simulink model "motorsPID"  (R2015a)
settings: Solver=ode45  StartTime=0.0  StopTime=Tsim  RelTol=1e-3
values from neighbouring files (symbols this model uses):
  b = 0.1    [AjusteC.m]    (also in AjusteC2.m; AjusteCVaryReal.m; GenPath.m = m*(2.0*pi/L); GenPath2.m = m*(2.0*pi/L))
  d = 0.4    [AjusteC.m]    (also in AjusteC2.m; AjusteCVaryReal.m; simula_robo.m)
  J = 0.01    [AjusteC.m]    (also in AjusteC2.m; AjusteCVaryReal.m; simula_robo.m)
  Kd = 0    [AjusteC.m]    (also in AjusteC2.m; AjusteCVaryReal.m; simula_robo.m)
  Ke = 0.08    [AjusteC.m]    (also in AjusteC2.m; AjusteCVaryReal.m; simula_robo.m)
  Ki = 10.0    (= 10)    [AjusteC.m]    (also in AjusteC2.m; AjusteCVaryReal.m; simula_robo.m)
  Kp = 5    [AjusteC.m]    (also in AjusteC2.m; AjusteCVaryReal.m; simula_robo.m)
  L = 0.5    [AjusteC.m]    (also in AjusteC2.m; AjusteCVaryReal.m; GenPath.m = input('Entre o comprimento m�ximo: '); GenPath2.m = input('Entre o comprimento m�ximo: '))
  Res = 1    [AjusteC.m]    (also in AjusteC2.m; AjusteCVaryReal.m; simula_robo.m)
  thetai = 0    [AjusteC.m]    (also in AjusteC2.m; AjusteCVaryReal.m; simula_robo.m = 1.57079632679)
  Ts = 0.1    [AjusteC.m]    (also in AjusteC2.m; AjusteCVaryReal.m; GenPath.m; GenPath2.m)
  vmax = 0.8    [AjusteC.m]    (also in AjusteC2.m; AjusteCVaryReal.m; simula_robo.m)
  vmin = -vmax    (= -0.8)    [AjusteC.m]    (also in AjusteC2.m; AjusteCVaryReal.m; simula_robo.m)
  wmax = 0.8    [AjusteC.m]    (also in AjusteC2.m; AjusteCVaryReal.m; simula_robo.m)
  wmin = -wmax    (= -0.8)    [AjusteC.m]    (also in AjusteC2.m; AjusteCVaryReal.m; simula_robo.m)
  xi = 0    [AjusteC.m]    (also in AjusteC2.m; AjusteCVaryReal.m = 1; simula_robo.m)
  yi = 0    [AjusteC.m]    (also in AjusteC2.m; AjusteCVaryReal.m = -3; simula_robo.m = -0.5)
libraries: simulink_extras x6, simulink x6
settings Model: Creator=Thiago  LastModifiedBy=Thiago

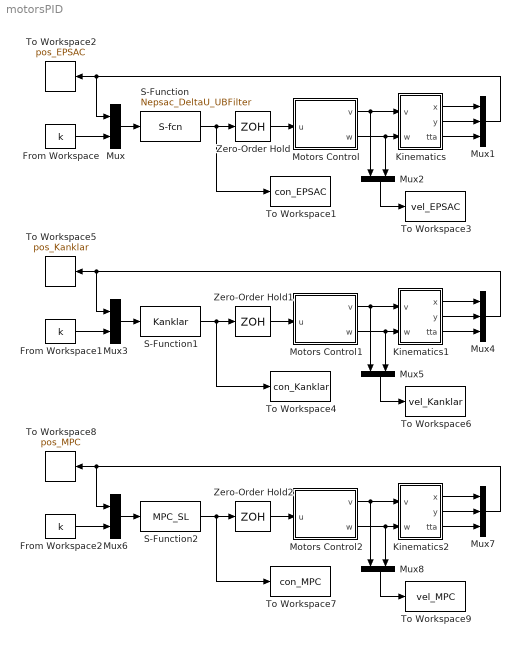
== system motorsPID ==
  From Workspace : FromWorkspace  VariableName=k  SampleTime=Ts
  From Workspace1 : FromWorkspace  VariableName=k  SampleTime=Ts
  From Workspace2 : FromWorkspace  VariableName=k  SampleTime=Ts
  Kinematics : Subsystem
  Kinematics1 : Subsystem
  Kinematics2 : Subsystem
  Motors Control : Subsystem
  Motors Control1 : Subsystem
  Motors Control2 : Subsystem
  Mux{,2..3,5..6,8} (6 alike) : Mux  Inputs=2
  Mux1 : Mux  Inputs=3
  Mux4 : Mux  Inputs=3
  Mux7 : Mux  Inputs=3
  S-Function : S-Function  FunctionName=Nepsac_DeltaU_UBFilter
  S-Function1 : S-Function  FunctionName=Kanklar
  S-Function2 : S-Function  FunctionName=MPC_SL
  To Workspace1 : ToWorkspace  VariableName=con_EPSAC  SaveFormat=Structure With Time  SampleTime=Ts
  To Workspace2 : ToWorkspace  VariableName=pos_EPSAC  SaveFormat=Structure With Time  SampleTime=Ts
  To Workspace3 : ToWorkspace  VariableName=vel_EPSAC  SaveFormat=Structure With Time  SampleTime=Ts
  To Workspace4 : ToWorkspace  VariableName=con_Kanklar  SaveFormat=Structure With Time  SampleTime=Ts
  To Workspace5 : ToWorkspace  VariableName=pos_Kanklar  SaveFormat=Structure With Time  SampleTime=Ts
  To Workspace6 : ToWorkspace  VariableName=vel_Kanklar  SaveFormat=Structure With Time  SampleTime=Ts
  To Workspace7 : ToWorkspace  VariableName=con_MPC  SaveFormat=Structure With Time  SampleTime=Ts
  To Workspace8 : ToWorkspace  VariableName=pos_MPC  SaveFormat=Structure With Time  SampleTime=Ts
  To Workspace9 : ToWorkspace  VariableName=vel_MPC  SaveFormat=Structure With Time  SampleTime=Ts
  Zero-Order Hold : ZeroOrderHold  SampleTime=Ts
  Zero-Order Hold1 : ZeroOrderHold  SampleTime=Ts
  Zero-Order Hold2 : ZeroOrderHold  SampleTime=Ts
  wires:
  S-Function/1 -> Zero-Order Hold/1, To Workspace1/1
  Motors Control/1(v) -> Kinematics/1(v), Mux2/1
  Motors Control/2(w) -> Kinematics/2(w), Mux2/2
  Kinematics/1(x) -> Mux1/1
  Kinematics/2(y) -> Mux1/2
  Kinematics/3(tta) -> Mux1/3
  Mux/1 -> S-Function/1
  From Workspace/1 -> Mux/2
  Mux1/1 -> Mux/1, To Workspace2/1
  Mux2/1 -> To Workspace3/1
  Zero-Order Hold/1 -> Motors Control/1(u)
  S-Function1/1 -> Zero-Order Hold1/1, To Workspace4/1
  Motors Control1/1(v) -> Kinematics1/1(v), Mux5/1
  Motors Control1/2(w) -> Kinematics1/2(w), Mux5/2
  Kinematics1/1(x) -> Mux4/1
  Kinematics1/2(y) -> Mux4/2
  Kinematics1/3(tta) -> Mux4/3
  Mux3/1 -> S-Function1/1
  From Workspace1/1 -> Mux3/2
  Mux4/1 -> Mux3/1, To Workspace5/1
  Mux5/1 -> To Workspace6/1
  Zero-Order Hold1/1 -> Motors Control1/1(u)
  S-Function2/1 -> Zero-Order Hold2/1, To Workspace7/1
  Motors Control2/1(v) -> Kinematics2/1(v), Mux8/1
  Motors Control2/2(w) -> Kinematics2/2(w), Mux8/2
  Kinematics2/1(x) -> Mux7/1
  Kinematics2/2(y) -> Mux7/2
  Kinematics2/3(tta) -> Mux7/3
  Mux6/1 -> S-Function2/1
  From Workspace2/1 -> Mux6/2
  Mux7/1 -> Mux6/1, To Workspace8/1
  Mux8/1 -> To Workspace9/1
  Zero-Order Hold2/1 -> Motors Control2/1(u)

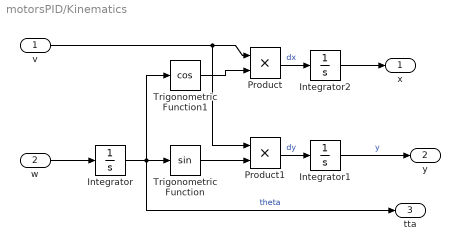
== system motorsPID/Kinematics ==
  v : Inport
  w : Inport  Port=2
  Integrator : Integrator  InitialCondition=thetai
  Integrator1 : Integrator  InitialCondition=yi
  Integrator2 : Integrator  InitialCondition=xi
  Product : Product
  Product1 : Product
  Trigonometric Function : Trigonometry
  Trigonometric Function1 : Trigonometry  Operator=cos
  x : Outport
  y : Outport  Port=2
  tta : Outport  Port=3
  wires:
  v/1 -> Product1/1, Product/1
  Trigonometric Function1/1 -> Product/2
  Product/1 -> Integrator2/1  "dx"
  Integrator/1 -> tta/1, Trigonometric Function1/1, Trigonometric Function/1  "theta"
  Integrator1/1 -> y/1  "y"
  Product1/1 -> Integrator1/1  "dy"
  Trigonometric Function/1 -> Product1/2
  Integrator2/1 -> x/1
  w/1 -> Integrator/1

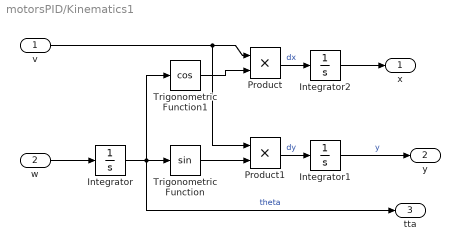
== system motorsPID/Kinematics1 ==
  v : Inport
  w : Inport  Port=2
  Integrator : Integrator  InitialCondition=thetai
  Integrator1 : Integrator  InitialCondition=yi
  Integrator2 : Integrator  InitialCondition=xi
  Product : Product
  Product1 : Product
  Trigonometric Function : Trigonometry
  Trigonometric Function1 : Trigonometry  Operator=cos
  x : Outport
  y : Outport  Port=2
  tta : Outport  Port=3
  wires:
  v/1 -> Product1/1, Product/1
  Trigonometric Function1/1 -> Product/2
  Product/1 -> Integrator2/1  "dx"
  Integrator/1 -> tta/1, Trigonometric Function1/1, Trigonometric Function/1  "theta"
  Integrator1/1 -> y/1  "y"
  Product1/1 -> Integrator1/1  "dy"
  Trigonometric Function/1 -> Product1/2
  Integrator2/1 -> x/1
  w/1 -> Integrator/1

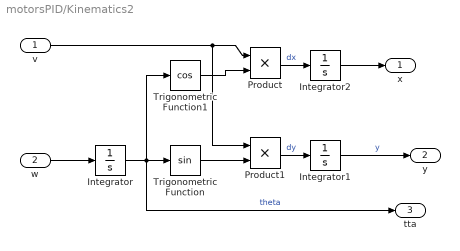
== system motorsPID/Kinematics2 ==
  v : Inport
  w : Inport  Port=2
  Integrator : Integrator  InitialCondition=thetai
  Integrator1 : Integrator  InitialCondition=yi
  Integrator2 : Integrator  InitialCondition=xi
  Product : Product
  Product1 : Product
  Trigonometric Function : Trigonometry
  Trigonometric Function1 : Trigonometry  Operator=cos
  x : Outport
  y : Outport  Port=2
  tta : Outport  Port=3
  wires:
  v/1 -> Product1/1, Product/1
  Trigonometric Function1/1 -> Product/2
  Product/1 -> Integrator2/1  "dx"
  Integrator/1 -> tta/1, Trigonometric Function1/1, Trigonometric Function/1  "theta"
  Integrator1/1 -> y/1  "y"
  Product1/1 -> Integrator1/1  "dy"
  Trigonometric Function/1 -> Product1/2
  Integrator2/1 -> x/1
  w/1 -> Integrator/1

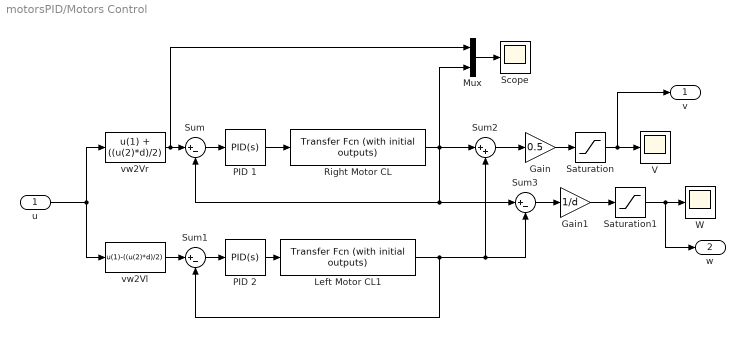
== system motorsPID/Motors Control ==
  u : Inport
  Gain : Gain  Gain=0.5
  Gain1 : Gain  Gain=1/d
  Left Motor CL1 : simulink_extras/Additional Linear/Transfer Fcn (with initial outputs)  N=[Ke]  D="[J*L  (J*Res+b*L) (b*Res+Ke^2)]"  Y0=0  U0=0
  Mux : Mux  Inputs=2
  PID 1 : simulink/Continuous/PID Controller  Controller=PID  TimeDomain=Continuous-time  SampleTime=-1  IntegratorMethod=Forward Euler  FilterMethod=Forward Euler  Form=Parallel  UseFilter=on  ControllerParametersSource=internal  P=Kp  I=Ki  D=Kd  N=100  InitialConditionSource=internal  InitialConditionForIntegrator=0  InitialConditionForFilter=0  ExternalReset=none  LimitOutput=off  UpperSaturationLimit=inf  LowerSaturationLimit=-inf  LinearizeAsGain=on  AntiWindupMode=none  Kb=1  TrackingMode=off  Kt=1  PParamMin=[]  PParamMax=[]  IParamMin=[]  IParamMax=[]  DParamMin=[]  DParamMax=[]  NParamMin=[]  NParamMax=[]  KbParamMin=[]  KbParamMax=[]  KtParamMin=[]  KtParamMax=[]  POutMin=[]  POutMax=[]  IOutMin=[]  IOutMax=[]  DOutMin=[]  DOutMax=[]  NOutMin=[]  NOutMax=[]  KbOutMin=[]  KbOutMax=[]  KtOutMin=[]  KtOutMax=[]  IntegratorOutMin=[]  IntegratorOutMax=[]  FilterOutMin=[]  FilterOutMax=[]  SumOutMin=[]  SumOutMax=[]  SumI1OutMin=[]  SumI1OutMax=[]  SumI2OutMin=[]  SumI2OutMax=[]  SumI3OutMin=[]  SumI3OutMax=[]  SumDOutMin=[]  SumDOutMax=[]  SaturationOutMin=[]  SaturationOutMax=[]  IntegratorContinuousStateAttributes=''  IntegratorStateMustResolveToSignalObject=off  IntegratorRTWStateStorageClass=Auto  FilterContinuousStateAttributes=''  FilterStateMustResolveToSignalObject=off  FilterRTWStateStorageClass=Auto  DifferentiatorICPrevScaledInput=0  DifferentiatorOutMin=[]  DifferentiatorOutMax=[]
  PID 2 : simulink/Continuous/PID Controller  Controller=PID  TimeDomain=Continuous-time  SampleTime=-1  IntegratorMethod=Forward Euler  FilterMethod=Forward Euler  Form=Parallel  UseFilter=on  ControllerParametersSource=internal  P=Kp  I=Ki  D=Kd  N=100  InitialConditionSource=internal  InitialConditionForIntegrator=0  InitialConditionForFilter=0  ExternalReset=none  LimitOutput=off  UpperSaturationLimit=inf  LowerSaturationLimit=-inf  LinearizeAsGain=on  AntiWindupMode=none  Kb=1  TrackingMode=off  Kt=1  PParamMin=[]  PParamMax=[]  IParamMin=[]  IParamMax=[]  DParamMin=[]  DParamMax=[]  NParamMin=[]  NParamMax=[]  KbParamMin=[]  KbParamMax=[]  KtParamMin=[]  KtParamMax=[]  POutMin=[]  POutMax=[]  IOutMin=[]  IOutMax=[]  DOutMin=[]  DOutMax=[]  NOutMin=[]  NOutMax=[]  KbOutMin=[]  KbOutMax=[]  KtOutMin=[]  KtOutMax=[]  IntegratorOutMin=[]  IntegratorOutMax=[]  FilterOutMin=[]  FilterOutMax=[]  SumOutMin=[]  SumOutMax=[]  SumI1OutMin=[]  SumI1OutMax=[]  SumI2OutMin=[]  SumI2OutMax=[]  SumI3OutMin=[]  SumI3OutMax=[]  SumDOutMin=[]  SumDOutMax=[]  SaturationOutMin=[]  SaturationOutMax=[]  IntegratorContinuousStateAttributes=''  IntegratorStateMustResolveToSignalObject=off  IntegratorRTWStateStorageClass=Auto  FilterContinuousStateAttributes=''  FilterStateMustResolveToSignalObject=off  FilterRTWStateStorageClass=Auto  DifferentiatorICPrevScaledInput=0  DifferentiatorOutMin=[]  DifferentiatorOutMax=[]
  Right Motor CL : simulink_extras/Additional Linear/Transfer Fcn (with initial outputs)  N=[Ke]  D="[J*L  (J*Res+b*L) (b*Res+Ke^2)]"  Y0=0  U0=0
  Saturation : Saturate  UpperLimit=vmax  LowerLimit=vmin
  Saturation1 : Saturate  UpperLimit=wmax  LowerLimit=wmin
  Scope : Scope
      settings: SaveName=ScopeData3
  Sum : Sum  Inputs=|+-
  Sum1 : Sum  Inputs=|+-
  Sum2 : Sum  Inputs=|++
  Sum3 : Sum  Inputs=|+-
  V : Scope
  W : Scope
      settings: SaveName=ScopeData2
  vw2Vl : Fcn  Expr=u(1)-((u(2)*d)/2)
  vw2Vr : Fcn  Expr=u(1) + ((u(2)*d)/2)
  v : Outport
  w : Outport  Port=2
  wires:
  u/1 -> vw2Vr/1, vw2Vl/1
  PID 1/1 -> Right Motor CL/1
  Sum/1 -> PID 1/1
  PID 2/1 -> Left Motor CL1/1
  Sum1/1 -> PID 2/1
  vw2Vl/1 -> Sum1/1
  Left Motor CL1/1 -> Sum3/2, Sum2/2, Sum1/2
  vw2Vr/1 -> Mux/1, Sum/1
  Right Motor CL/1 -> Mux/2, Sum2/1, Sum3/1, Sum/2
  Sum2/1 -> Gain/1
  Sum3/1 -> Gain1/1
  Mux/1 -> Scope/1
  Gain/1 -> Saturation/1
  Saturation/1 -> v/1, V/1
  Gain1/1 -> Saturation1/1
  Saturation1/1 -> W/1, w/1

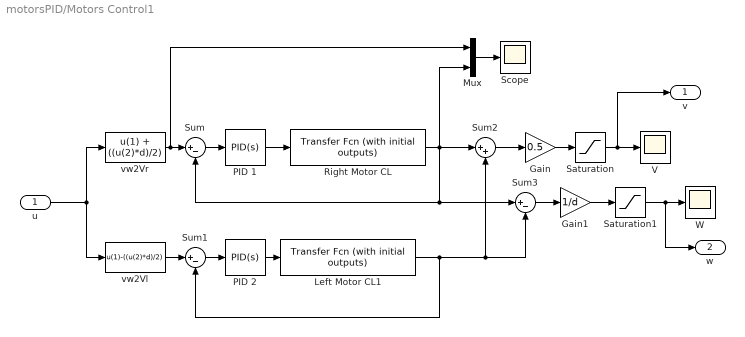
== system motorsPID/Motors Control1 ==
  u : Inport
  Gain : Gain  Gain=0.5
  Gain1 : Gain  Gain=1/d
  Left Motor CL1 : simulink_extras/Additional Linear/Transfer Fcn (with initial outputs)  N=[Ke]  D="[J*L  (J*Res+b*L) (b*Res+Ke^2)]"  Y0=0  U0=0
  Mux : Mux  Inputs=2
  PID 1 : simulink/Continuous/PID Controller  Controller=PID  TimeDomain=Continuous-time  SampleTime=-1  IntegratorMethod=Forward Euler  FilterMethod=Forward Euler  Form=Parallel  UseFilter=on  ControllerParametersSource=internal  P=Kp  I=Ki  D=Kd  N=100  InitialConditionSource=internal  InitialConditionForIntegrator=0  InitialConditionForFilter=0  ExternalReset=none  LimitOutput=off  UpperSaturationLimit=inf  LowerSaturationLimit=-inf  LinearizeAsGain=on  AntiWindupMode=none  Kb=1  TrackingMode=off  Kt=1  PParamMin=[]  PParamMax=[]  IParamMin=[]  IParamMax=[]  DParamMin=[]  DParamMax=[]  NParamMin=[]  NParamMax=[]  KbParamMin=[]  KbParamMax=[]  KtParamMin=[]  KtParamMax=[]  POutMin=[]  POutMax=[]  IOutMin=[]  IOutMax=[]  DOutMin=[]  DOutMax=[]  NOutMin=[]  NOutMax=[]  KbOutMin=[]  KbOutMax=[]  KtOutMin=[]  KtOutMax=[]  IntegratorOutMin=[]  IntegratorOutMax=[]  FilterOutMin=[]  FilterOutMax=[]  SumOutMin=[]  SumOutMax=[]  SumI1OutMin=[]  SumI1OutMax=[]  SumI2OutMin=[]  SumI2OutMax=[]  SumI3OutMin=[]  SumI3OutMax=[]  SumDOutMin=[]  SumDOutMax=[]  SaturationOutMin=[]  SaturationOutMax=[]  IntegratorContinuousStateAttributes=''  IntegratorStateMustResolveToSignalObject=off  IntegratorRTWStateStorageClass=Auto  FilterContinuousStateAttributes=''  FilterStateMustResolveToSignalObject=off  FilterRTWStateStorageClass=Auto  DifferentiatorICPrevScaledInput=0  DifferentiatorOutMin=[]  DifferentiatorOutMax=[]
  PID 2 : simulink/Continuous/PID Controller  Controller=PID  TimeDomain=Continuous-time  SampleTime=-1  IntegratorMethod=Forward Euler  FilterMethod=Forward Euler  Form=Parallel  UseFilter=on  ControllerParametersSource=internal  P=Kp  I=Ki  D=Kd  N=100  InitialConditionSource=internal  InitialConditionForIntegrator=0  InitialConditionForFilter=0  ExternalReset=none  LimitOutput=off  UpperSaturationLimit=inf  LowerSaturationLimit=-inf  LinearizeAsGain=on  AntiWindupMode=none  Kb=1  TrackingMode=off  Kt=1  PParamMin=[]  PParamMax=[]  IParamMin=[]  IParamMax=[]  DParamMin=[]  DParamMax=[]  NParamMin=[]  NParamMax=[]  KbParamMin=[]  KbParamMax=[]  KtParamMin=[]  KtParamMax=[]  POutMin=[]  POutMax=[]  IOutMin=[]  IOutMax=[]  DOutMin=[]  DOutMax=[]  NOutMin=[]  NOutMax=[]  KbOutMin=[]  KbOutMax=[]  KtOutMin=[]  KtOutMax=[]  IntegratorOutMin=[]  IntegratorOutMax=[]  FilterOutMin=[]  FilterOutMax=[]  SumOutMin=[]  SumOutMax=[]  SumI1OutMin=[]  SumI1OutMax=[]  SumI2OutMin=[]  SumI2OutMax=[]  SumI3OutMin=[]  SumI3OutMax=[]  SumDOutMin=[]  SumDOutMax=[]  SaturationOutMin=[]  SaturationOutMax=[]  IntegratorContinuousStateAttributes=''  IntegratorStateMustResolveToSignalObject=off  IntegratorRTWStateStorageClass=Auto  FilterContinuousStateAttributes=''  FilterStateMustResolveToSignalObject=off  FilterRTWStateStorageClass=Auto  DifferentiatorICPrevScaledInput=0  DifferentiatorOutMin=[]  DifferentiatorOutMax=[]
  Right Motor CL : simulink_extras/Additional Linear/Transfer Fcn (with initial outputs)  N=[Ke]  D="[J*L  (J*Res+b*L) (b*Res+Ke^2)]"  Y0=0  U0=0
  Saturation : Saturate  UpperLimit=vmax  LowerLimit=vmin
  Saturation1 : Saturate  UpperLimit=wmax  LowerLimit=wmin
  Scope : Scope
      settings: SaveName=ScopeData3
  Sum : Sum  Inputs=|+-
  Sum1 : Sum  Inputs=|+-
  Sum2 : Sum  Inputs=|++
  Sum3 : Sum  Inputs=|+-
  V : Scope
  W : Scope
      settings: SaveName=ScopeData2
  vw2Vl : Fcn  Expr=u(1)-((u(2)*d)/2)
  vw2Vr : Fcn  Expr=u(1) + ((u(2)*d)/2)
  v : Outport
  w : Outport  Port=2
  wires:
  u/1 -> vw2Vr/1, vw2Vl/1
  PID 1/1 -> Right Motor CL/1
  Sum/1 -> PID 1/1
  PID 2/1 -> Left Motor CL1/1
  Sum1/1 -> PID 2/1
  vw2Vl/1 -> Sum1/1
  Left Motor CL1/1 -> Sum3/2, Sum2/2, Sum1/2
  vw2Vr/1 -> Mux/1, Sum/1
  Right Motor CL/1 -> Mux/2, Sum2/1, Sum3/1, Sum/2
  Sum2/1 -> Gain/1
  Sum3/1 -> Gain1/1
  Mux/1 -> Scope/1
  Gain/1 -> Saturation/1
  Saturation/1 -> v/1, V/1
  Gain1/1 -> Saturation1/1
  Saturation1/1 -> W/1, w/1

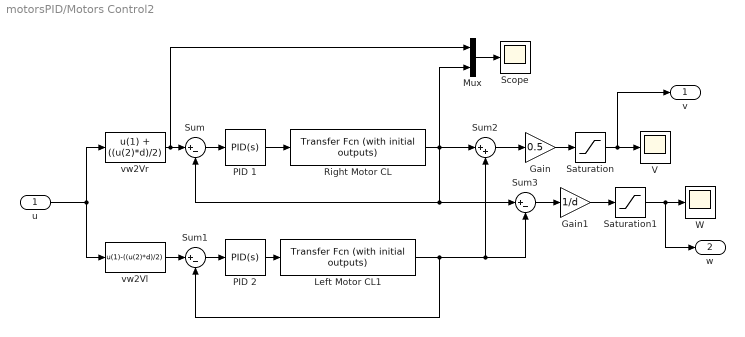
== system motorsPID/Motors Control2 ==
  u : Inport
  Gain : Gain  Gain=0.5
  Gain1 : Gain  Gain=1/d
  Left Motor CL1 : simulink_extras/Additional Linear/Transfer Fcn (with initial outputs)  N=[Ke]  D="[J*L  (J*Res+b*L) (b*Res+Ke^2)]"  Y0=0  U0=0
  Mux : Mux  Inputs=2
  PID 1 : simulink/Continuous/PID Controller  Controller=PID  TimeDomain=Continuous-time  SampleTime=-1  IntegratorMethod=Forward Euler  FilterMethod=Forward Euler  Form=Parallel  UseFilter=on  ControllerParametersSource=internal  P=Kp  I=Ki  D=Kd  N=100  InitialConditionSource=internal  InitialConditionForIntegrator=0  InitialConditionForFilter=0  ExternalReset=none  LimitOutput=off  UpperSaturationLimit=inf  LowerSaturationLimit=-inf  LinearizeAsGain=on  AntiWindupMode=none  Kb=1  TrackingMode=off  Kt=1  PParamMin=[]  PParamMax=[]  IParamMin=[]  IParamMax=[]  DParamMin=[]  DParamMax=[]  NParamMin=[]  NParamMax=[]  KbParamMin=[]  KbParamMax=[]  KtParamMin=[]  KtParamMax=[]  POutMin=[]  POutMax=[]  IOutMin=[]  IOutMax=[]  DOutMin=[]  DOutMax=[]  NOutMin=[]  NOutMax=[]  KbOutMin=[]  KbOutMax=[]  KtOutMin=[]  KtOutMax=[]  IntegratorOutMin=[]  IntegratorOutMax=[]  FilterOutMin=[]  FilterOutMax=[]  SumOutMin=[]  SumOutMax=[]  SumI1OutMin=[]  SumI1OutMax=[]  SumI2OutMin=[]  SumI2OutMax=[]  SumI3OutMin=[]  SumI3OutMax=[]  SumDOutMin=[]  SumDOutMax=[]  SaturationOutMin=[]  SaturationOutMax=[]  IntegratorContinuousStateAttributes=''  IntegratorStateMustResolveToSignalObject=off  IntegratorRTWStateStorageClass=Auto  FilterContinuousStateAttributes=''  FilterStateMustResolveToSignalObject=off  FilterRTWStateStorageClass=Auto  DifferentiatorICPrevScaledInput=0  DifferentiatorOutMin=[]  DifferentiatorOutMax=[]
  PID 2 : simulink/Continuous/PID Controller  Controller=PID  TimeDomain=Continuous-time  SampleTime=-1  IntegratorMethod=Forward Euler  FilterMethod=Forward Euler  Form=Parallel  UseFilter=on  ControllerParametersSource=internal  P=Kp  I=Ki  D=Kd  N=100  InitialConditionSource=internal  InitialConditionForIntegrator=0  InitialConditionForFilter=0  ExternalReset=none  LimitOutput=off  UpperSaturationLimit=inf  LowerSaturationLimit=-inf  LinearizeAsGain=on  AntiWindupMode=none  Kb=1  TrackingMode=off  Kt=1  PParamMin=[]  PParamMax=[]  IParamMin=[]  IParamMax=[]  DParamMin=[]  DParamMax=[]  NParamMin=[]  NParamMax=[]  KbParamMin=[]  KbParamMax=[]  KtParamMin=[]  KtParamMax=[]  POutMin=[]  POutMax=[]  IOutMin=[]  IOutMax=[]  DOutMin=[]  DOutMax=[]  NOutMin=[]  NOutMax=[]  KbOutMin=[]  KbOutMax=[]  KtOutMin=[]  KtOutMax=[]  IntegratorOutMin=[]  IntegratorOutMax=[]  FilterOutMin=[]  FilterOutMax=[]  SumOutMin=[]  SumOutMax=[]  SumI1OutMin=[]  SumI1OutMax=[]  SumI2OutMin=[]  SumI2OutMax=[]  SumI3OutMin=[]  SumI3OutMax=[]  SumDOutMin=[]  SumDOutMax=[]  SaturationOutMin=[]  SaturationOutMax=[]  IntegratorContinuousStateAttributes=''  IntegratorStateMustResolveToSignalObject=off  IntegratorRTWStateStorageClass=Auto  FilterContinuousStateAttributes=''  FilterStateMustResolveToSignalObject=off  FilterRTWStateStorageClass=Auto  DifferentiatorICPrevScaledInput=0  DifferentiatorOutMin=[]  DifferentiatorOutMax=[]
  Right Motor CL : simulink_extras/Additional Linear/Transfer Fcn (with initial outputs)  N=[Ke]  D="[J*L  (J*Res+b*L) (b*Res+Ke^2)]"  Y0=0  U0=0
  Saturation : Saturate  UpperLimit=vmax  LowerLimit=vmin
  Saturation1 : Saturate  UpperLimit=wmax  LowerLimit=wmin
  Scope : Scope
      settings: SaveName=ScopeData3
  Sum : Sum  Inputs=|+-
  Sum1 : Sum  Inputs=|+-
  Sum2 : Sum  Inputs=|++
  Sum3 : Sum  Inputs=|+-
  V : Scope
  W : Scope
      settings: SaveName=ScopeData2
  vw2Vl : Fcn  Expr=u(1)-((u(2)*d)/2)
  vw2Vr : Fcn  Expr=u(1) + ((u(2)*d)/2)
  v : Outport
  w : Outport  Port=2
  wires:
  u/1 -> vw2Vr/1, vw2Vl/1
  PID 1/1 -> Right Motor CL/1
  Sum/1 -> PID 1/1
  PID 2/1 -> Left Motor CL1/1
  Sum1/1 -> PID 2/1
  vw2Vl/1 -> Sum1/1
  Left Motor CL1/1 -> Sum3/2, Sum2/2, Sum1/2
  vw2Vr/1 -> Mux/1, Sum/1
  Right Motor CL/1 -> Mux/2, Sum2/1, Sum3/1, Sum/2
  Sum2/1 -> Gain/1
  Sum3/1 -> Gain1/1
  Mux/1 -> Scope/1
  Gain/1 -> Saturation/1
  Saturation/1 -> v/1, V/1
  Gain1/1 -> Saturation1/1
  Saturation1/1 -> W/1, w/1
